simulink model "RCAMDemoMinimal_Model"  (R2024b)
settings: Solver=VariableStepAuto  StartTime=0.0  StopTime=10.0  RelTol=1e-3
values from neighbouring files (symbols this model uses):
  u1max = 25*pi/180    (= 0.436332312999)    [RCAM_model.m]
  u1min = -25*pi/180    (= -0.436332312999)    [RCAM_model.m]
  u2max = 10*pi/180    (= 0.174532925199)    [RCAM_model.m]
  u2min = -25*pi/180    (= -0.436332312999)    [RCAM_model.m]
  u3max = 30*pi/180    (= 0.523598775598)    [RCAM_model.m]
  u3min = - 30*pi/180    (= -0.523598775598)    [RCAM_model.m]
  u4max = 10*pi/180    (= 0.174532925199)    [RCAM_model.m]
  u5max = 10*pi/180    (= 0.174532925199)    [RCAM_model.m]
  u5min = 0.5*pi/180    (= 0.00872664625997)    [RCAM_model.m]
  Uo = [ ... (first row only)    [LineariseSymmetricDifferences.m]
  x0 = [85 ... (first row only)    [sim_initialise.m]
undefined symbols (not defined in the file or in its folder): RCAM_model_new, u14min
libraries: aeroblk_lib_HL20 x4, aerolibanimutils x2
settings Model: Creator=satvik_sh  LastModifiedBy=satvik_sh

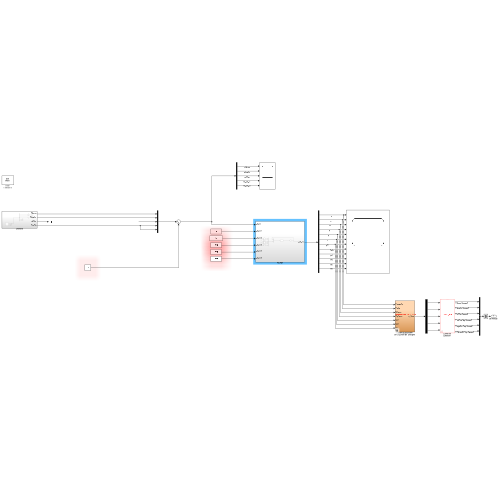
[thumbnail: Simulink's stored preview of the top-level diagram]
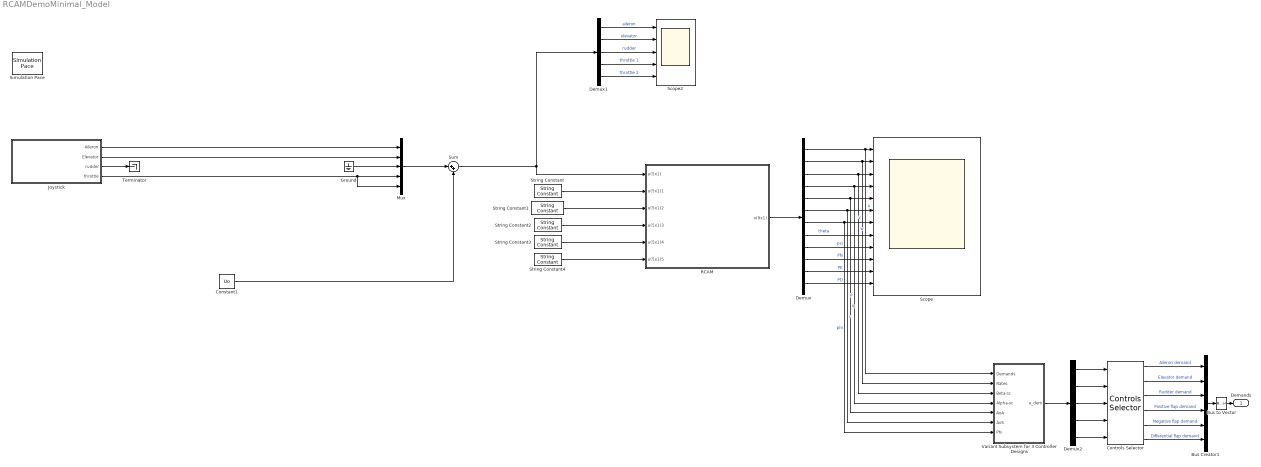
== system RCAMDemoMinimal_Model ==
  Bus Creator1 : BusCreator  Inputs=6
  Bus to Vector : BusToVector
  Constant1 : Constant  Value=Uo
  Controls Selector : aeroblk_lib_HL20/Controls Selector  SystemSampleTime=-1  SSRTWFcnClass=[]  VariantActivationTime=update diagram  AllowFlexibleInterface=on  Latency=0  AutoFrameSizeCalculation=off
  Demux : Demux  Outputs=12
  Demux1 : Demux  Outputs=5
  Demux2 : Demux  Outputs=5
  Ground : Ground
  Joystick : Subsystem
  Mux : Mux  Inputs=5
  RCAM : Subsystem
  Scope : Scope  NumInputPorts=12
  Scope2 : Scope  NumInputPorts=5
  Simulation Pace : aerolibanimutils/Simulation Pace  SimulationPace=1  SleepMode=Auto  OutputPaceError=off  SampleTime=1/30
  String Constant : StringConstant  String=g
  String Constant1 : StringConstant  String=rho
  String Constant2 : StringConstant  String=Xcg
  String Constant3 : StringConstant  String=Ycg
  String Constant4 : StringConstant  String=Zcg
  Sum : Sum  Inputs=|++
  Terminator : Terminator
  Variant Subsystem for 3 Controller Designs : Subsystem  Variant=on  VariantControlMode=label  LabelModeActiveChoice=ClassicalController
  Demands : Outport  VectorParamsAs1DForOutWhenUnconnected=off
  wires:
  Demux/8 -> Scope/8  "theta"
  Demux/10 -> Scope/10  "PN"
  Demux/1 -> Variant Subsystem for 3 Controller Designs/1(Demands), Scope/1  "u"
  RCAM/1(x(9x1)) -> Demux/1
  String Constant3/1 -> RCAM/5(u(5x1)4)
  String Constant2/1 -> RCAM/4(u(5x1)3)
  String Constant4/1 -> RCAM/6(u(5x1)5)
  String Constant/1 -> RCAM/2(u(5x1)1)
  String Constant1/1 -> RCAM/3(u(5x1)2)
  Demux/11 -> Scope/11  "PE"
  Demux/9 -> Scope/9  "psi"
  Demux/12 -> Scope/12  "PD"
  Demux1/4 -> Scope2/4  "throttle 1"
  Demux1/3 -> Scope2/3  "rudder"
  Demux/7 -> Variant Subsystem for 3 Controller Designs/7(Phi), Scope/7  "phi"
  Demux/4 -> Variant Subsystem for 3 Controller Designs/4(Alpha-sc), Scope/4  "p"
  Demux/6 -> Variant Subsystem for 3 Controller Designs/6(AoS), Scope/6  "r"
  Demux1/1 -> Scope2/1  "aileron"
  Demux/5 -> Variant Subsystem for 3 Controller Designs/5(AoA), Scope/5  "q"
  Demux/3 -> Variant Subsystem for 3 Controller Designs/3(Beta-sc), Scope/3  "w"
  Demux1/2 -> Scope2/2  "elevator"
  Demux/2 -> Variant Subsystem for 3 Controller Designs/2(Rates), Scope/2  "v"
  Sum/1 -> Demux1/1, RCAM/1(u(5x1))
  Demux1/5 -> Scope2/5  "throttle 2"
  Mux/1 -> Sum/1
  Joystick/1(Aileron) -> Mux/1
  Joystick/2(Elevator) -> Mux/2
  Joystick/3(rudder) -> Terminator/1
  Ground/1 -> Mux/3
  Joystick/4(throttle) -> Mux/5, Mux/4
  Constant1/1 -> Sum/2
  Variant Subsystem for 3 Controller Designs/1(u_dem) -> Demux2/1
  Bus to Vector/1 -> Demands/1
  Controls Selector/1 -> Bus Creator1/1  "Aileron demand"
  Controls Selector/4 -> Bus Creator1/4  "Positive flap demand"
  Controls Selector/2 -> Bus Creator1/2  "Elevator demand"
  Controls Selector/5 -> Bus Creator1/5  "Negative flap demand"
  Bus Creator1/1 -> Bus to Vector/1
  Controls Selector/3 -> Bus Creator1/3  "Rudder demand"
  Controls Selector/6 -> Bus Creator1/6  "Differential flap demand"
  Demux2/1 -> Controls Selector/1
  Demux2/2 -> Controls Selector/2
  Demux2/3 -> Controls Selector/3
  Demux2/4 -> Controls Selector/4
  Demux2/5 -> Controls Selector/5

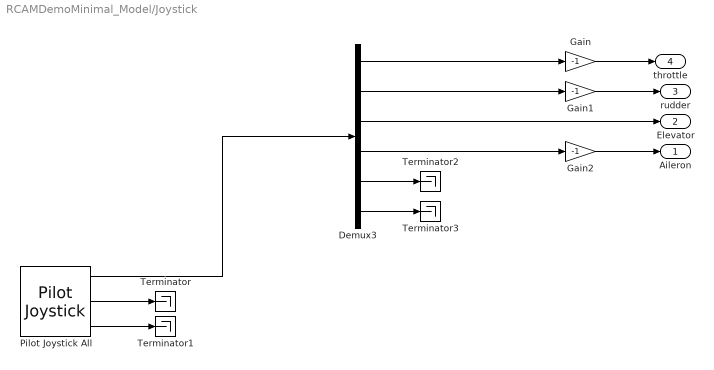
== system RCAMDemoMinimal_Model/Joystick ==
  Demux3 : Demux  Outputs=6
  Gain : Gain  Gain=-1
  Gain1 : Gain  Gain=-1
  Gain2 : Gain  Gain=-1
  Pilot Joystick All : aerolibanimutils/Pilot Joystick  JoystickID=Joystick1  OutputConfiguration=AllOutputs  SampleTime=1/30
      settings: LibrarySourceBlock=aerolibanimutils/Pilot Joystick All
  Terminator{,1..3} (4 alike) : Terminator
  Aileron : Outport
  Elevator : Outport  Port=2
  rudder : Outport  Port=3
  throttle : Outport  Port=4
  wires:
  Demux3/4 -> Gain2/1
  Gain2/1 -> Aileron/1
  Pilot Joystick All/1 -> Demux3/1
  Demux3/2 -> Gain1/1
  Demux3/5 -> Terminator2/1
  Gain1/1 -> rudder/1
  Pilot Joystick All/3 -> Terminator1/1
  Demux3/3 -> Elevator/1
  Gain/1 -> throttle/1
  Pilot Joystick All/2 -> Terminator/1
  Demux3/1 -> Gain/1
  Demux3/6 -> Terminator3/1

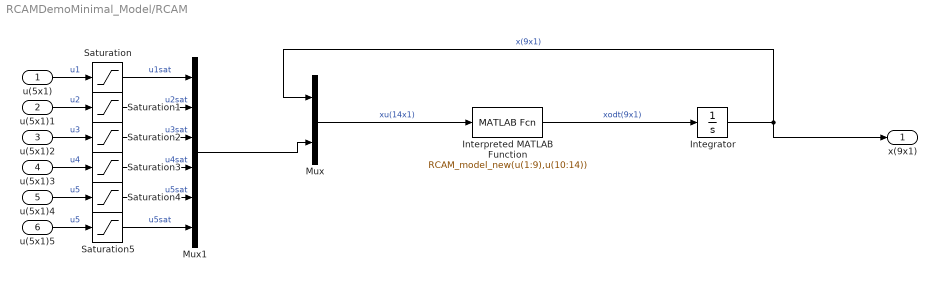
== system RCAMDemoMinimal_Model/RCAM ==
  u(5x1) : Inport
  u(5x1)1 : Inport  Port=2
  u(5x1)2 : Inport  Port=3
  u(5x1)3 : Inport  Port=4
  u(5x1)4 : Inport  Port=5
  u(5x1)5 : Inport  Port=6
  Integrator : Integrator  InitialCondition=x0
  Interpreted MATLAB Function : MATLABFcn  MATLABFcn=RCAM_model_new(u(1:9),u(10:14))
  Mux : Mux  Inputs=2
  Mux1 : Mux  Inputs=6
  Saturation : Saturate  UpperLimit=u1max  LowerLimit=u1min
  Saturation1 : Saturate  UpperLimit=u2max  LowerLimit=u2min
  Saturation2 : Saturate  UpperLimit=u3max  LowerLimit=u3min
  Saturation3 : Saturate  UpperLimit=u4max  LowerLimit=u14min
  Saturation4 : Saturate  UpperLimit=u5max  LowerLimit=u5min
  Saturation5 : Saturate  UpperLimit=u5max  LowerLimit=u5min
  x(9x1) : Outport
  wires:
  Interpreted MATLAB Function/1 -> Integrator/1  "xodt(9x1)"
  Mux/1 -> Interpreted MATLAB Function/1  "xu(14x1)"
  Integrator/1 -> x(9x1)/1, Mux/1  "x(9x1)"
  u(5x1)/1 -> Saturation/1  "u1"
  u(5x1)1/1 -> Saturation1/1  "u2"
  u(5x1)2/1 -> Saturation2/1  "u3"
  u(5x1)3/1 -> Saturation3/1  "u4"
  u(5x1)4/1 -> Saturation4/1  "u5"
  Saturation/1 -> Mux1/1  "u1sat"
  Saturation1/1 -> Mux1/2  "u2sat"
  Saturation2/1 -> Mux1/3  "u3sat"
  Saturation3/1 -> Mux1/4  "u4sat"
  Saturation4/1 -> Mux1/5  "u5sat"
  Mux1/1 -> Mux/2
  u(5x1)5/1 -> Saturation5/1  "u5"
  Saturation5/1 -> Mux1/6  "u5sat"

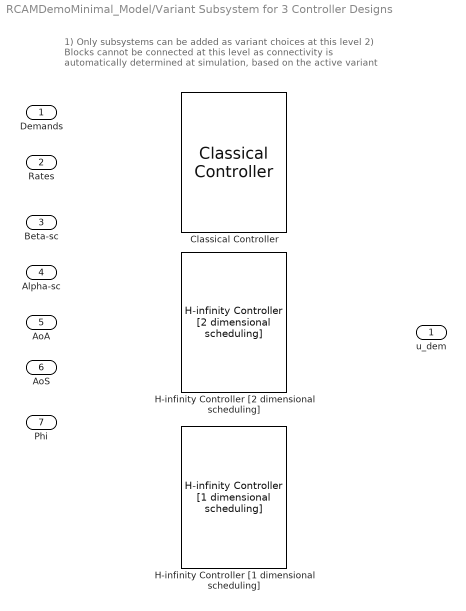
== system RCAMDemoMinimal_Model/Variant Subsystem for 3 Controller Designs ==
  note: 1) Only subsystems can be added as variant choices at this level
      | 2) Blocks cannot be connected at this level as connectivity is
      | automatically determined at simulation, based on the active variant
  Demands : Inport
  Rates : Inport  Port=2
  Beta-sc : Inport  Port=3
  Alpha-sc : Inport  Port=4
  AoA : Inport  Port=5
  AoS : Inport  Port=6
  Phi : Inport  Port=7
  Classical Controller : aeroblk_lib_HL20/Classical Controller  SystemSampleTime=-1  SSRTWFcnClass=[]  VariantControl=ClassicalController  VariantActivationTime=update diagram  AllowFlexibleInterface=on  Latency=0  AutoFrameSizeCalculation=off
  H-infinity Controller [1 dimensional scheduling] : aeroblk_lib_HL20/H-infinity Controller [1 dimensional scheduling]  SystemSampleTime=-1  VariantControl=HInf1DimensionalController  VariantActivationTime=update diagram  AllowFlexibleInterface=on  Latency=0  AutoFrameSizeCalculation=off
  H-infinity Controller [2 dimensional scheduling] : aeroblk_lib_HL20/H-infinity Controller [2 dimensional scheduling]  SystemSampleTime=-1  VariantControl=HInf2DimensionalController  VariantActivationTime=update diagram  AllowFlexibleInterface=on  Latency=0  AutoFrameSizeCalculation=off
  u_dem : Outport  VectorParamsAs1DForOutWhenUnconnected=off
